simulink model "RSCodingErasuresPunctShortExample"  (R2014a)
settings: Solver=FixedStepDiscrete  StartTime=0.0  StopTime=inf  RelTol=1e-3
PreLoadFcn:
  | RS_TsUncoded = 1;   % Sample time
  | RS_n = 63;  % Codeword length
  | RS_k = 53;  % Message length
  | RS_shortenLength = 35;  % Shortening length
  | RS_numPuncs = 2;  % Number of punctures
  | RS_MQAM = 64;  % QAM order
  | RS_EbNoUncoded = 15;  % In dB
  | RS_EbNoCoded = RS_EbNoUncoded + 10*log10( (RS_k - RS_shortenLength) / (RS_n - RS_shortenLength - RS_numPuncs) );  % Eb/No of coded signal, in dB
  | RS_numBitsPerSymbol = log2(RS_MQAM);  % 6 bits per symbol
  | RS_sigPower = 42;  % Assume points at +/-1, +/-3, +/-5, +/-7, +/-9
  | RS_TsymCoded = RS_TsUncoded * (RS_k - RS_shortenLength) / (RS_n - RS_shortenLength - RS_numPuncs);  % Symbol time of coded signal
  | RS_numErasures = 6;
InitFcn:
  | RS_TsUncoded = 1;   % Sample time
  | RS_n = 63;  % Codeword length
  | RS_k = 53;  % Message length
  | RS_shortenLength = 35;  % Shortening length
  | RS_numPuncs = 2;  % Number of punctures
  | RS_MQAM = 64;  % QAM order
  | RS_EbNoUncoded = 15;  % In dB
  | RS_EbNoCoded = RS_EbNoUncoded + 10*log10( (RS_k - RS_shortenLength) / (RS_n - RS_shortenLength - RS_numPuncs) );  % Eb/No of coded signal, in dB
  | RS_numBitsPerSymbol = log2(RS_MQAM);  % 6 bits per symbol
  | RS_sigPower = 42;  % Assume points at +/-1, +/-3, +/-5, +/-7, +/-9
  | RS_TsymCoded = RS_TsUncoded * (RS_k - RS_shortenLength) / (RS_n - RS_shortenLength - RS_numPuncs);  % Symbol time of coded signal
  | RS_numErasures = 6;
undefined symbols (not defined in the file or in its folder): commblksprivate, Info, rsgenpoly
libraries: commutil2 x4, commdigbbndam3 x2, commsink2 x2, commblkcod2 x2, commchan3 x1, dspstat3 x1, dspmathops x1, commrandsrc2 x1
Description:
  | Shortened Reed-Solomon Coding with Erasures and Punctures
settings Model: ExtModeAutoUpdateStatusClock=off  Creator=The MathWorks Inc.
settings DataIOCC: SaveFormat=Structure  SignalLoggingSaveFormat=ModelDataLogs  SaveOutput=off  SignalLogging=off
settings OptimizationCC: ExpressionDepthLimit=2147483647  InitFltsAndDblsToZero=on  EfficientMapNaN2IntZero=off
settings DebuggingCC: UnderspecifiedInitializationDetection=Classic  SolverPrmCheckMsg=none  FcnCallInpInsideContextMsg=UseLocalSettings  StrictBusMsg=Warning
settings GRTTargetCC: TargetFcnLib=ansi_tfl_tmw_new.mat  CombineOutputUpdateFcns=off  GRTInterface=on

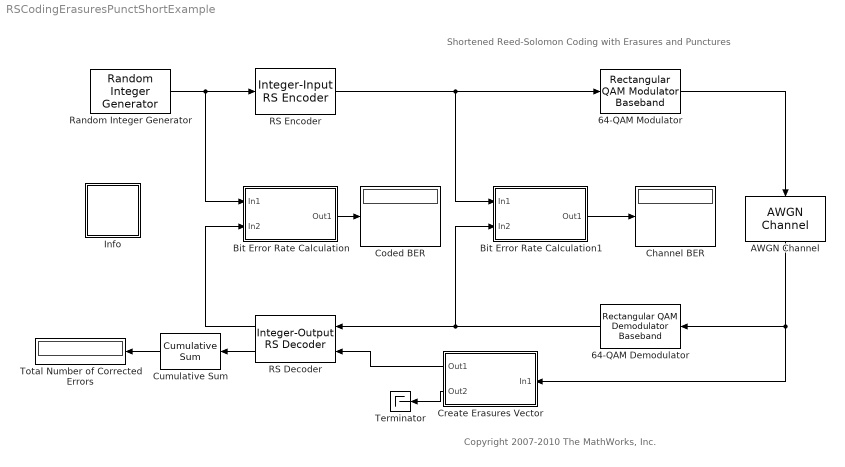
== system RSCodingErasuresPunctShortExample ==
  note: Shortened Reed-Solomon Coding with Erasures and Punctures
  note: Copyright 2007-2010 The MathWorks, Inc.
  64-QAM Demodulator : commdigbbndam3/Rectangular QAM Demodulator Baseband  M=RS_MQAM  PowType=Min. distance between symbols  MinDist=2  AvgPow=1  PeakPow=1  Ph=0  Dec=Gray  Mapping=[0:15]  OutType=Integer  DecType=Hard decision  VarSource=Dialog  Variance=1  outDtype1=Inherit via internal rule  outDtype2=Inherit via internal rule  derotateFactorWordLen=16  denormFactorWordLen=16  prodOutWordLen=32  prodOutRoundingMode=Floor  prodOutOverflowMode=Wrap  sumWordLen=32
  64-QAM Modulator : commdigbbndam3/Rectangular QAM Modulator Baseband  M=RS_MQAM  InType=Integer  Enc=Gray  Mapping=[0:15]  PowType=Min. distance between symbols  MinDist=2  AvgPow=1  PeakPow=1  Ph=0  outDtype=double  outWordLen=16  outUDDataType=sfix(16)  outFracLenMode=Best precision  outFracLen=15
  AWGN Channel : commchan3/AWGN Channel  InputProcessing=Columns as channels (frame based)  seed=67  noiseMode="Signal to noise ratio  (Eb/No)"  EbNodB="RS_EbNoCoded  % RS_EbNoUncoded + 10*log10( (RS_k - RS_shortenLength) / (RS_n - RS_shortenLength - RS_numPuncs) )"  EsNodB=10  SNRdB=10  bitsPerSym=RS_numBitsPerSymbol  Ps=RS_sigPower  Tsym="RS_TsymCoded  % RS_TsUncoded * (RS_k - RS_shortenLength) / (RS_n - RS_shortenLength - RS_numPuncs)"  variance=1
  Bit Error Rate Calculation : Subsystem
      mask Display:
      | disp('Bit Error\nRate\nCalculation')
      | port_label('input', 1, 'Tx')
      | port_label('input', 2, 'Rx')
  Bit Error Rate Calculation1 : Subsystem
      mask Display:
      | disp('Bit Error\nRate\nCalculation')
      | port_label('input', 1, 'Tx')
      | port_label('input', 2, 'Rx')
  Channel BER : Display
  Coded BER : Display
  Create Erasures Vector : Subsystem
      mask Display:
      | disp('Create\nErasures\nVector')
      | port_label('output', 1, 'era')
      | port_label('output', 2, 'eSig')
  Cumulative Sum : dspmathops/Cumulative Sum  dim=Channels (running sum)  InputProcessing=Columns as channels (frame based)  reset_popup=None  outputDataTypeStr=Inherit: Same as accumulator  outputLastDataTypeStr=Inherit: Same as accumulator  outputMin=[]  outputMax=[]  roundingMode=Floor  overflowMode=off
  Info : Subsystem  AncestorBlock=commblksprivate/Info  mask(Info){}
      settings: OpenFcn=helpview([docroot '/toolbox/comm/comm.map'], 'doc_rs_shortened')
      mask Display: disp('Info')
  RS Decoder : commblkcod2/Integer-Output RS Decoder  n=RS_n - RS_shortenLength  k=RS_k - RS_shortenLength  specPrimPoly=on  prPoly=de2bi(primpoly(6, 'nodisplay'), 'left-msb')  specGenPoly=off  genPoly=rsgenpoly(7,3)  specPuncture=on  punctVec=[ones(RS_n - RS_k - RS_numPuncs,1); zeros(RS_numPuncs,1)]  specErasurePort=on  showNumErr=on
  RS Encoder : commblkcod2/Integer-Input RS Encoder  n=RS_n - RS_shortenLength  k=RS_k - RS_shortenLength  specPrimPoly=on  prPoly=de2bi(primpoly(6, 'nodisplay'), 'left-msb')  specGenPoly=off  genPoly=rsgenpoly(7,3)  specPuncture=on  punctVec=[ones(RS_n - RS_k - RS_numPuncs,1); zeros(RS_numPuncs,1)]
  Random Integer Generator : commrandsrc2/Random Integer Generator  mul=RS_MQAM  seed=37  Ts=RS_TsUncoded  frameBased=on  sampPerFrame=RS_k - RS_shortenLength  orient=off  outDataType=double
  Terminator : Terminator
  Total Number of Corrected Errors : Display
  wires:
  Random Integer Generator/1 -> RS Encoder/1, Bit Error Rate Calculation/1(In1)
  RS Encoder/1 -> 64-QAM Modulator/1, Bit Error Rate Calculation1/1(In1)
  64-QAM Modulator/1 -> AWGN Channel/1
  AWGN Channel/1 -> 64-QAM Demodulator/1, Create Erasures Vector/1(In1)
  64-QAM Demodulator/1 -> RS Decoder/1, Bit Error Rate Calculation1/2(In2)
  RS Decoder/1 -> Bit Error Rate Calculation/2(In2)
  Bit Error Rate Calculation/1(Out1) -> Coded BER/1
  Create Erasures Vector/1(Out1) -> RS Decoder/2
  Bit Error Rate Calculation1/1(Out1) -> Channel BER/1
  RS Decoder/2 -> Cumulative Sum/1
  Cumulative Sum/1 -> Total Number of Corrected Errors/1
  Create Erasures Vector/2(Out2) -> Terminator/1

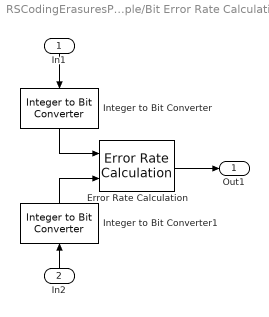
== system RSCodingErasuresPunctShortExample/Bit Error Rate Calculation ==
  In1 : Inport
  In2 : Inport  Port=2
  Error Rate Calculation : commsink2/Error Rate Calculation  N=0  st_delay=0  cp_mode=Entire frame  subframe=[]  PMode=Port  WsName=ErrorVec  RsMode2=off  stop=on  numErr=1000  maxBits=1e8
  Integer to Bit Converter : commutil2/Integer to Bit Converter  nbits=6  signedInputValues=Unsigned  bitOrder=MSB first  outDtype=Inherit via internal rule
  Integer to Bit Converter1 : commutil2/Integer to Bit Converter  nbits=6  signedInputValues=Unsigned  bitOrder=MSB first  outDtype=Inherit via internal rule
  Out1 : Outport
  wires:
  Integer to Bit Converter/1 -> Error Rate Calculation/1
  Integer to Bit Converter1/1 -> Error Rate Calculation/2
  In1/1 -> Integer to Bit Converter/1
  Error Rate Calculation/1 -> Out1/1
  In2/1 -> Integer to Bit Converter1/1

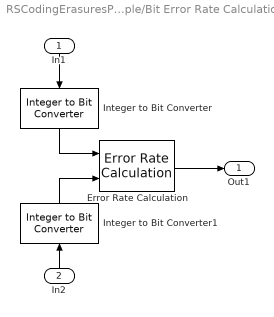
== system RSCodingErasuresPunctShortExample/Bit Error Rate Calculation1 ==
  In1 : Inport
  In2 : Inport  Port=2
  Error Rate Calculation : commsink2/Error Rate Calculation  N=0  st_delay=0  cp_mode=Entire frame  subframe=[]  PMode=Port  WsName=ErrorVec  RsMode2=off  stop=off  numErr=100  maxBits=1e6
  Integer to Bit Converter : commutil2/Integer to Bit Converter  nbits=6  signedInputValues=Unsigned  bitOrder=MSB first  outDtype=Inherit via internal rule
  Integer to Bit Converter1 : commutil2/Integer to Bit Converter  nbits=6  signedInputValues=Unsigned  bitOrder=MSB first  outDtype=Inherit via internal rule
  Out1 : Outport
  wires:
  In2/1 -> Integer to Bit Converter1/1
  Error Rate Calculation/1 -> Out1/1
  In1/1 -> Integer to Bit Converter/1
  Integer to Bit Converter1/1 -> Error Rate Calculation/2
  Integer to Bit Converter/1 -> Error Rate Calculation/1

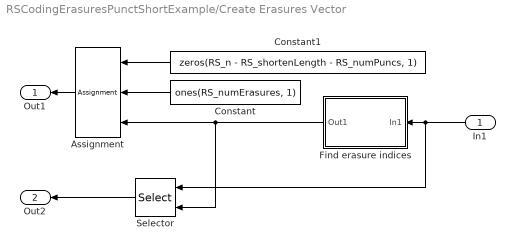
== system RSCodingErasuresPunctShortExample/Create Erasures Vector ==
  In1 : Inport
  Assignment : Assignment  NumberOfDimensions=2  IndexOptions=Index vector (port),Index vector (dialog)  Indices=1,1  OutputSizes=1,1
  Constant : Constant  Value=ones(RS_numErasures, 1)  VectorParams1D=off  FramePeriod=RS_TsUncoded * (RS_k - RS_shortenLength)
      settings: SamplingMode=Frame based
  Constant1 : Constant  Value=zeros(RS_n - RS_shortenLength - RS_numPuncs, 1)  VectorParams1D=off  FramePeriod=RS_TsUncoded * (RS_k - RS_shortenLength)
      settings: SamplingMode=Frame based
  Find erasure indices : Subsystem
      mask Display:
      | port_label('output', 1, 'idx')
      | disp('Find\nerasure\nindices')
  Selector : Selector  NumberOfDimensions=2  InputPortWidth=3  IndexOptions=Index vector (port),Index vector (dialog)  Indices=[1 3],1  OutputSizes=1,1
  Out1 : Outport
  Out2 : Outport  Port=2
  wires:
  Find erasure indices/1(Out1) -> Assignment/3, Selector/2
  Constant/1 -> Assignment/2
  Constant1/1 -> Assignment/1
  In1/1 -> Find erasure indices/1(In1), Selector/1
  Assignment/1 -> Out1/1
  Selector/1 -> Out2/1

== system RSCodingErasuresPunctShortExample/Info ==

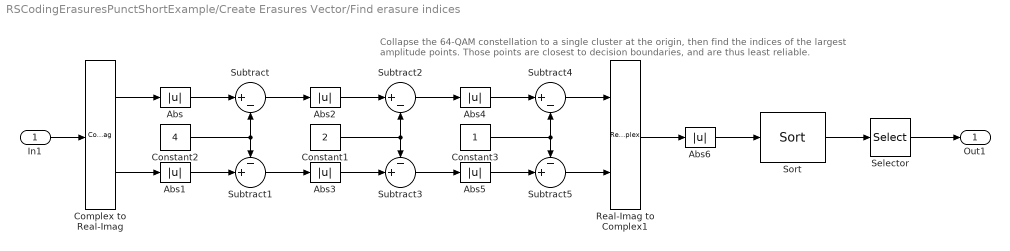
== system RSCodingErasuresPunctShortExample/Create Erasures Vector/Find erasure indices ==
  note: Collapse the 64-QAM constellation to a single cluster at the origin, then find the indices of the largest amplitude points.
      | Those points are closest to decision boundaries, and are thus least reliable.
  In1 : Inport
  Abs{,1..6} (7 alike) : Abs
  Complex to Real-Imag : ComplexToRealImag
  Constant1 : Constant  Value=2  VectorParams1D=off  FramePeriod=RS_TsUncoded * (RS_k - RS_shortenLength)
      settings: SamplingMode=Frame based
  Constant2 : Constant  Value=4  VectorParams1D=off  FramePeriod=RS_TsUncoded * (RS_k - RS_shortenLength)
      settings: SamplingMode=Frame based
  Constant3 : Constant  VectorParams1D=off  FramePeriod=RS_TsUncoded * (RS_k - RS_shortenLength)
      settings: SamplingMode=Frame based
  Real-Imag to Complex1 : RealImagToComplex
  Selector : Selector  NumberOfDimensions=2  InputPortWidth=3  IndexOptions=Index vector (dialog),Index vector (dialog)  Indices=[63-35-6-2+1:63-35-2],1  OutputSizes=1,1
  Sort : dspstat3/Sort  otype=Index  dir=Ascending  sortAlg=Quick sort  accumDataTypeStr=Inherit: Same as product output  accumLastDataTypeStr=Inherit: Same as product output  roundingMode=Floor  overflowMode=off
  Subtract : Sum  Inputs=|+-
  Subtract1 : Sum  Inputs=-+|
  Subtract2 : Sum  Inputs=|+-
  Subtract3 : Sum  Inputs=-+|
  Subtract4 : Sum  Inputs=|+-
  Subtract5 : Sum  Inputs=-+|
  Out1 : Outport
  wires:
  Complex to Real-Imag/1 -> Abs/1
  Complex to Real-Imag/2 -> Abs1/1
  Abs/1 -> Subtract/1
  Constant2/1 -> Subtract/2, Subtract1/1
  Abs1/1 -> Subtract1/2
  Subtract/1 -> Abs2/1
  Subtract1/1 -> Abs3/1
  Abs2/1 -> Subtract2/1
  Abs3/1 -> Subtract3/2
  Constant1/1 -> Subtract2/2, Subtract3/1
  Subtract2/1 -> Abs4/1
  Subtract3/1 -> Abs5/1
  Abs4/1 -> Subtract4/1
  Abs5/1 -> Subtract5/2
  Constant3/1 -> Subtract4/2, Subtract5/1
  Subtract4/1 -> Real-Imag to Complex1/1
  Subtract5/1 -> Real-Imag to Complex1/2
  Real-Imag to Complex1/1 -> Abs6/1
  Abs6/1 -> Sort/1
  In1/1 -> Complex to Real-Imag/1
  Sort/1 -> Selector/1
  Selector/1 -> Out1/1
